simulink model "Modell_PID"  (R2023a)
settings: Solver=FixedStepAuto  StartTime=0.0  StopTime=479  FixedStep=1/30  RelTol=1e-3
undefined symbols (not defined in the file): DiscIntNeverNeededParam, dsys, w
libraries: slident x2, simulink x1
settings Model: Creator=Legenden-PC  LastModifiedBy=Legenden-PC
settings OptimizationCC: ReuseModelBlockBuffer=off

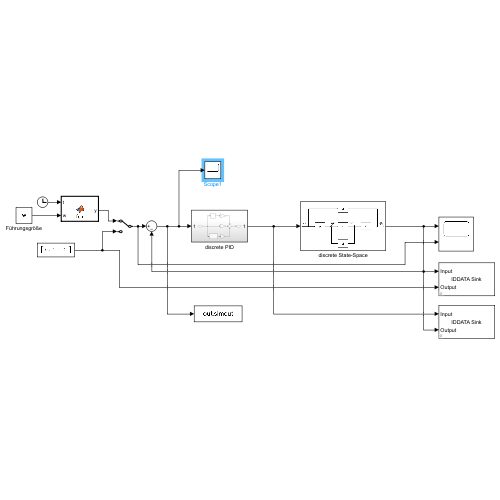
[thumbnail: Simulink's stored preview of the top-level diagram]
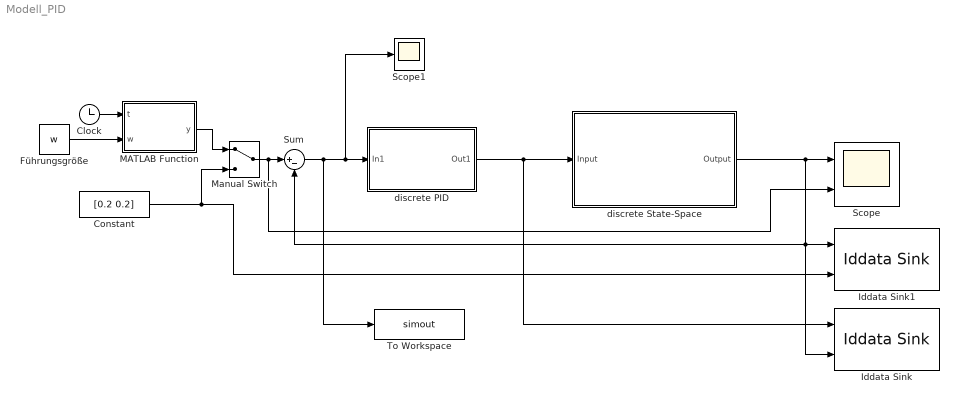
== system Modell_PID ==
  Clock : Clock
  Constant : Constant  Value=[0.2 0.2]
  Führungsgröße : Constant  Value=w  SampleTime=1/30
  Iddata Sink : slident/Iddata Sink  datasetname=ymodel  Ts=1/30  isu=on  isy=on
  Iddata Sink1 : slident/Iddata Sink  datasetname=w_vs_model  Ts=1/30  isu=on  isy=on
  MATLAB Function : MATLAB Function  TreatAsAtomicUnit=on
  Manual Switch : ManualSwitch
  Scope : Scope  NumInputPorts=2
  Scope1 : Scope
  Sum : Sum  Inputs=|+-
  To Workspace : ToWorkspace  VariableName=simout  SaveFormat=Timeseries  SampleTime=-1
  discrete PID : Subsystem
  discrete State-Space : Subsystem
      mask Display: image('$imagefile'); % Use "Edit Image" on toolstrip to change.
  wires:
  discrete State-Space/1(Output) -> Sum/2, Iddata Sink1/1, Iddata Sink/2, Scope/1
  Sum/1 -> To Workspace/1, Scope1/1, discrete PID/1(In1)
  discrete PID/1(Out1) -> Iddata Sink/1, discrete State-Space/1(Input)
  Clock/1 -> MATLAB Function/1(t)
  Führungsgröße/1 -> MATLAB Function/2(w)
  Constant/1 -> Manual Switch/2, Iddata Sink1/2
  Manual Switch/1 -> Scope/2, Sum/1
  MATLAB Function/1(y) -> Manual Switch/1

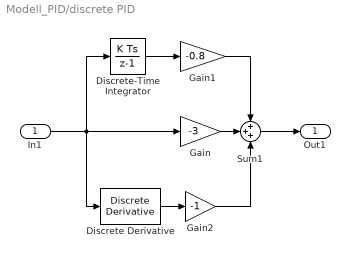
== system Modell_PID/discrete PID ==
  In1 : Inport
  Discrete Derivative : simulink/Discrete/Discrete Derivative  gainval=1.0  ICPrevScaledInput=0.0  OutMin=[]  OutMax=[]  OutDataType=fixdt(1, 16)  OutScaling=2^-10  DoSatur=off
  Discrete-Time Integrator : DiscreteIntegrator  SampleTime=1/30  ICPrevOutput=DiscIntNeverNeededParam  ICPrevScaledInput=DiscIntNeverNeededParam
  Gain : Gain  Gain=-3
  Gain1 : Gain  Gain=-0.8
  Gain2 : Gain  Gain=-1
  Sum1 : Sum  Inputs=+++
  Out1 : Outport
  wires:
  Gain/1 -> Sum1/2
  Gain2/1 -> Sum1/3
  Discrete Derivative/1 -> Gain2/1
  In1/1 -> Discrete Derivative/1, Discrete-Time Integrator/1, Gain/1
  Discrete-Time Integrator/1 -> Gain1/1
  Gain1/1 -> Sum1/1
  Sum1/1 -> Out1/1

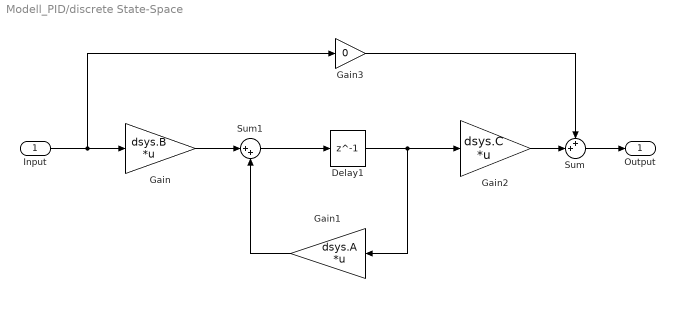
== system Modell_PID/discrete State-Space ==
  Input : Inport
  Delay1 : Delay  DelayLength=1  InitialCondition=[w(1,1) 0 w(1,2) 0]'
  Gain : Gain  Gain=dsys.B  Multiplication=Matrix(K*u)
  Gain1 : Gain  Gain=dsys.A  Multiplication=Matrix(K*u)
  Gain2 : Gain  Gain=dsys.C  Multiplication=Matrix(K*u)
  Gain3 : Gain  Gain=0
  Sum : Sum  Inputs=++|
  Sum1 : Sum  Inputs=|++
  Output : Outport
  wires:
  Input/1 -> Gain3/1, Gain/1
  Gain/1 -> Sum1/1
  Sum1/1 -> Delay1/1
  Delay1/1 -> Gain1/1, Gain2/1
  Gain1/1 -> Sum1/2
  Gain2/1 -> Sum/2
  Gain3/1 -> Sum/1
  Sum/1 -> Output/1

== matlab function Modell_PID/MATLAB Function ==
  data: t input; y output; w input
function y = fcn(t,w)

persistent k

if isempty(k)
    k=0;
end

%alle 5 Sekunden
if(mod(t,5)==0)
    k=k+1;
end

if k>size(w,1)
    k = size(w,1)
end

y = w(k,:)';
